simulink library "INT_WESDem_CalcState"  (R2016b)
settings: Solver=VariableStepAuto  StartTime=0.0  StopTime=10.0  RelTol=1e-3
settings Model: Creator=zhoukai  LastModifiedBy=zhoukai

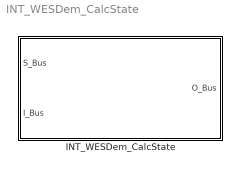
== system INT_WESDem_CalcState ==
  INT_WESDem_CalcState : Subsystem

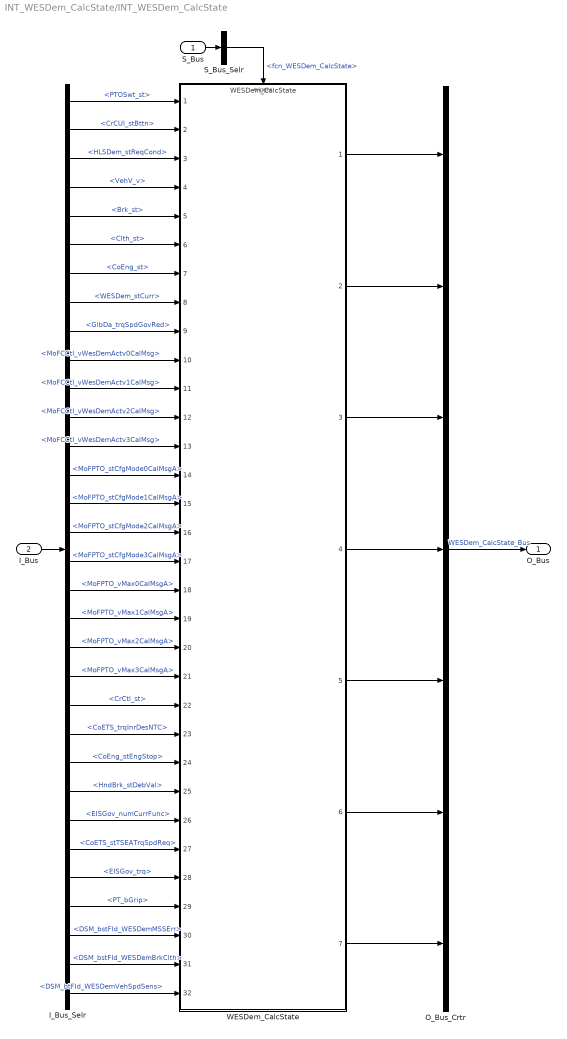
== system INT_WESDem_CalcState/INT_WESDem_CalcState ==
  S_Bus : Inport
  I_Bus : Inport  Port=2
  I_Bus_Selr : BusSelector  OutputSignals=PTOSwt_st,CrCUI_stBttn,HLSDem_stReqCond,VehV_v,Brk_st,Clth_st,CoEng_st,WESDem_stCurr,GlbDa_trqSpdGovRed,MoFCCtl_vWesDemActv0CalMsg,MoFCCtl_vWesDemActv1CalMsg,MoFCCtl_vWesDemActv2CalMsg,MoFCCtl_vWesDemActv3CalMsg,MoFPTO_stCfgMode0CalMsgA,MoFPTO_stCfgMode1CalMsgA,MoFPTO_stCfgMode2CalMsgA,MoFPTO_stCfgMode3CalMsgA,MoFPTO_vMax0CalMsgA,MoFPTO_vMax1CalMsgA,MoFPTO_vMax2CalMsgA,MoFPTO_vMax3CalMsgA,CrCtl_st,CoETS_trqInrDesNTC,CoEng_stEngStop,HndBrk_stDebVal,EISGov_numCurrFunc,CoETS_stTSEATrqSpdReq,EISGov_trq,PT_bGrip,DSM_bstFId_WESDemMSSErr,DSM_bstFId_WESDemBrkClth,DSM_btFId_WESDemVehSpdSens
  O_Bus_Crtr : BusCreator  Inputs=7
  S_Bus_Selr : BusSelector  OutputSignals=fcn_WESDem_CalcState
  WESDem_CalcState : ModelReference  ModelNameDialog=WESDem_CalcState  SimulationMode=Normal  ModelReferenceVersion=1.157  TriggerPortName=function  TriggerPortTriggerType=function-call  TriggerPortStatesWhenEnabling=held
  O_Bus : Outport
  wires:
  S_Bus_Selr/1 -> WESDem_CalcState/Trigger  "<fcn_WESDem_CalcState>"
  S_Bus/1 -> S_Bus_Selr/1
  I_Bus/1 -> I_Bus_Selr/1
  I_Bus_Selr/1 -> WESDem_CalcState/1  "<PTOSwt_st>"
  I_Bus_Selr/2 -> WESDem_CalcState/2  "<CrCUI_stBttn>"
  I_Bus_Selr/3 -> WESDem_CalcState/3  "<HLSDem_stReqCond>"
  I_Bus_Selr/4 -> WESDem_CalcState/4  "<VehV_v>"
  I_Bus_Selr/5 -> WESDem_CalcState/5  "<Brk_st>"
  I_Bus_Selr/6 -> WESDem_CalcState/6  "<Clth_st>"
  I_Bus_Selr/7 -> WESDem_CalcState/7  "<CoEng_st>"
  I_Bus_Selr/8 -> WESDem_CalcState/8  "<WESDem_stCurr>"
  I_Bus_Selr/9 -> WESDem_CalcState/9  "<GlbDa_trqSpdGovRed>"
  I_Bus_Selr/10 -> WESDem_CalcState/10  "<MoFCCtl_vWesDemActv0CalMsg>"
  I_Bus_Selr/11 -> WESDem_CalcState/11  "<MoFCCtl_vWesDemActv1CalMsg>"
  I_Bus_Selr/12 -> WESDem_CalcState/12  "<MoFCCtl_vWesDemActv2CalMsg>"
  I_Bus_Selr/13 -> WESDem_CalcState/13  "<MoFCCtl_vWesDemActv3CalMsg>"
  I_Bus_Selr/14 -> WESDem_CalcState/14  "<MoFPTO_stCfgMode0CalMsgA>"
  I_Bus_Selr/15 -> WESDem_CalcState/15  "<MoFPTO_stCfgMode1CalMsgA>"
  I_Bus_Selr/16 -> WESDem_CalcState/16  "<MoFPTO_stCfgMode2CalMsgA>"
  I_Bus_Selr/17 -> WESDem_CalcState/17  "<MoFPTO_stCfgMode3CalMsgA>"
  I_Bus_Selr/18 -> WESDem_CalcState/18  "<MoFPTO_vMax0CalMsgA>"
  I_Bus_Selr/19 -> WESDem_CalcState/19  "<MoFPTO_vMax1CalMsgA>"
  I_Bus_Selr/20 -> WESDem_CalcState/20  "<MoFPTO_vMax2CalMsgA>"
  I_Bus_Selr/21 -> WESDem_CalcState/21  "<MoFPTO_vMax3CalMsgA>"
  I_Bus_Selr/22 -> WESDem_CalcState/22  "<CrCtl_st>"
  I_Bus_Selr/23 -> WESDem_CalcState/23  "<CoETS_trqInrDesNTC>"
  I_Bus_Selr/24 -> WESDem_CalcState/24  "<CoEng_stEngStop>"
  I_Bus_Selr/25 -> WESDem_CalcState/25  "<HndBrk_stDebVal>"
  I_Bus_Selr/26 -> WESDem_CalcState/26  "<EISGov_numCurrFunc>"
  I_Bus_Selr/27 -> WESDem_CalcState/27  "<CoETS_stTSEATrqSpdReq>"
  I_Bus_Selr/28 -> WESDem_CalcState/28  "<EISGov_trq>"
  I_Bus_Selr/29 -> WESDem_CalcState/29  "<PT_bGrip>"
  I_Bus_Selr/30 -> WESDem_CalcState/30  "<DSM_bstFId_WESDemMSSErr>"
  I_Bus_Selr/31 -> WESDem_CalcState/31  "<DSM_bstFId_WESDemBrkClth>"
  I_Bus_Selr/32 -> WESDem_CalcState/32  "<DSM_btFId_WESDemVehSpdSens>"
  O_Bus_Crtr/1 -> O_Bus/1  "WESDem_CalcState_Bus"
  WESDem_CalcState/1 -> O_Bus_Crtr/1
  WESDem_CalcState/2 -> O_Bus_Crtr/2
  WESDem_CalcState/3 -> O_Bus_Crtr/3
  WESDem_CalcState/4 -> O_Bus_Crtr/4
  WESDem_CalcState/5 -> O_Bus_Crtr/5
  WESDem_CalcState/6 -> O_Bus_Crtr/6
  WESDem_CalcState/7 -> O_Bus_Crtr/7
